simulink model "example26"  (R2023b)
settings: Solver=VariableStepAuto  StartTime=0.0  StopTime=10.0  RelTol=1e-3
settings Model: Creator=ray  LastModifiedBy=ray

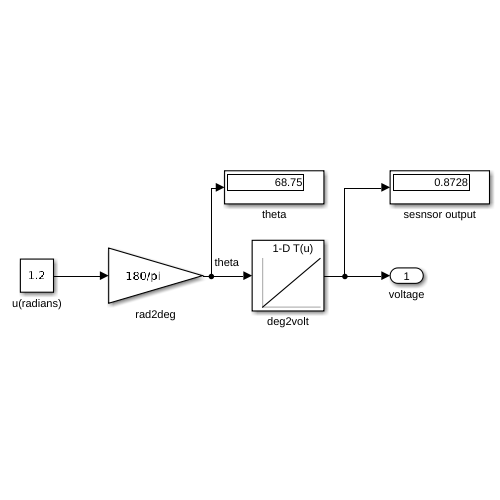
[thumbnail: Simulink's stored preview of the top-level diagram]
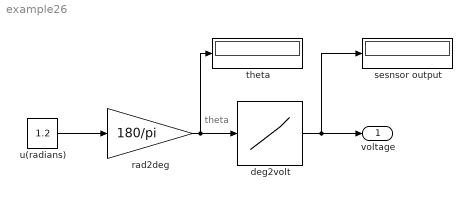
== system example26 ==
  note: theta
  deg2volt : Lookup_n-D  NumberOfTableDimensions=1  BreakpointsForDimension1=[0 90]  Table=tanh([0.5 4.5])  ExtrapMethod=Clip  InternalRulePriority=Speed  RndMeth=Simplest
  rad2deg : Gain  Gain=180/pi
  sesnsor output : Display
  theta : Display
  u(radians) : Constant  Value=1.2
  voltage : Outport
  wires:
  u(radians)/1 -> rad2deg/1
  rad2deg/1 -> theta/1, deg2volt/1
  deg2volt/1 -> sesnsor output/1, voltage/1
